simulink model "SineWave"  (R2015b)
settings: Solver=VariableStepAuto  StartTime=0.0  StopTime=10.0  RelTol=1e-3
StartFcn:
  | open_scope
settings Model: Creator=LUBO  LastModifiedBy=LUBO
settings OptimizationCC: BlockReduction=off  DefaultParameterBehavior=Inlined  BufferReuse=off

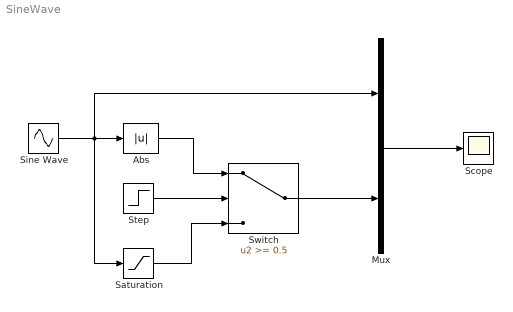
== system SineWave ==
  Abs : Abs
  Mux : Mux  Inputs=2
  Saturation : Saturate
  Scope : Scope
  Sine Wave : Sin  Phase=[0.2 0.5]  SampleTime=0
  Step : Step  Time=5  Before=1  After=0  SampleTime=0
  Switch : Switch  Threshold=0.5
  wires:
  Sine Wave/1 -> Saturation/1, Mux/1, Abs/1
  Saturation/1 -> Switch/3
  Abs/1 -> Switch/1
  Switch/1 -> Mux/2
  Mux/1 -> Scope/1
  Step/1 -> Switch/2
